simulink model "bounding_spine_Physical"  (R2024a)
settings: Solver=FixedStepDiscrete  StartTime=0.0  StopTime=inf  RelTol=1e-3  EnableMultiTasking=on
InitFcn:
  | run('initBusObjects.m')
  | run('parameters.m')
model workspace (MAT data in the model file):
  omega = 8
  zeta = 0.05
libraries: aru_toolbox x1
settings Model: SimulationMode=external  Creator=Mechatronics  LastModifiedBy=heath
settings SolverCC: ConcurrentTasks=on  AlgebraicLoopSolver=TrustRegion  PositivePriorityOrder=on  InsertRTBMode=Never (minimum delay)
settings DataIOCC: SaveFormat=Array  SaveState=on  SignalLoggingName=logsOut
settings OptimizationCC: BlockReduction=off  BooleanDataType=off  OptimizeBlockIOStorage=off  BufferReuse=off  GlobalBufferReuse=off  ExpressionFolding=off  LocalBlockOutputs=off  InitFltsAndDblsToZero=on  OptimizeDataStoreBuffers=off  BusAssignmentInplaceUpdate=off
settings DebuggingCC: SaveWithParameterizedLinksMsg=none  UnderspecifiedInitializationDetection=Classic  MergeDetectMultiDrivingBlocksExec=none  CheckExecutionContextPreStartOutputMsg=on  SignalResolutionControl=TryResolveAllWithWarning  TasksWithSamePriorityMsg=none  UnconnectedInputMsg=warning  UnconnectedOutputMsg=warning  UnconnectedLineMsg=warning  SFUnexpectedBacktrackingDiag=warning  SFNoUnconditionalDefaultTransitionDiag=warning  SFExecutionAtInitializationDiag=none  ArithmeticOperatorsInVariantConditions=warning
settings HardwareCC: ProdBitPerLong=64  ProdLongLongMode=on  ProdHWDeviceType=Intel->x86-64 (Linux 64)
settings ModelReferenceCC: EnableRefExpFcnMdlSchedulingChecks=on  PropagateSignalLabelsOutOfModel=off
settings SFSimCC: SimUseLocalCustomCode=off  SimTargetLang=C++
settings RTWCC: Description=Speedgoat Real-Time Target Machine  SystemTargetFile=speedgoat.tlc  TemplateMakefile=slrealtime_default_tmf  RTWUseLocalCustomCode=off  Toolchain=Simulink Real-Time Toolchain  BuildConfiguration=Faster Runs  CodeExecutionProfiling=on  TargetLang=C++  GPUComputeCapability=3.5  DLArmComputeVersion=19.05
settings CodeAppCC: StateflowObjectComments=on
settings SimulinkRealTimeTargetCC: InstructionSetFMA=off  LogToMDFFile=off
settings ConfigComp: CovMetricSettings=dw  CovSaveCumulativeToWorkspaceVar=on  CovSaveSingleToWorkspaceVar=on  CovExternalEMLEnable=off  CovSFcnEnable=off

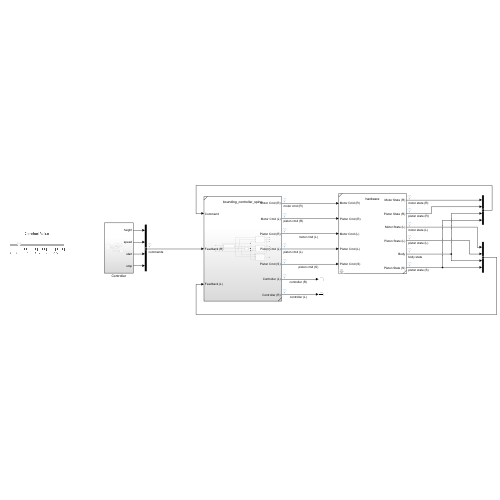
[thumbnail: Simulink's stored preview of the top-level diagram]
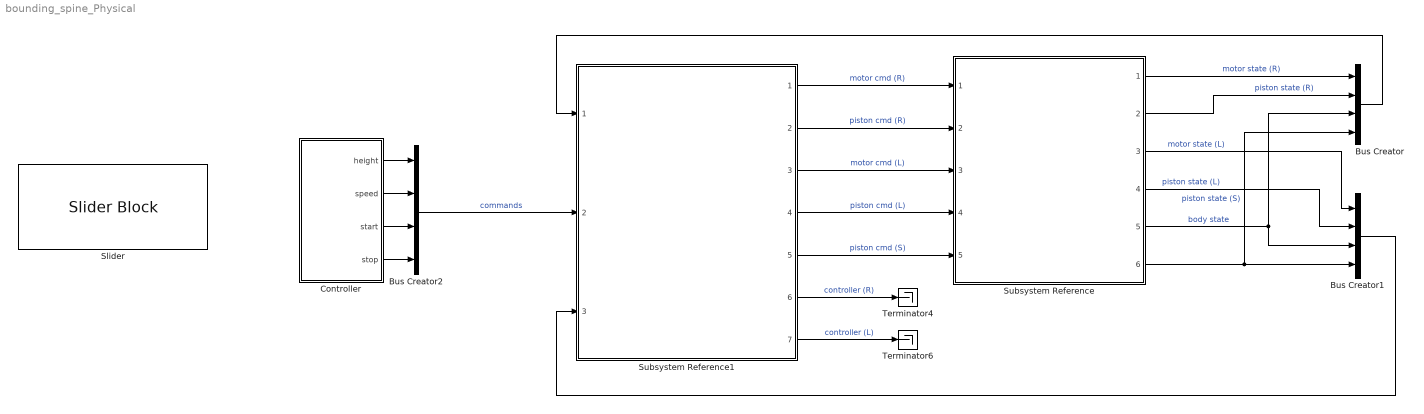
== system bounding_spine_Physical ==
  Bus Creator : BusCreator  Inputs=4  OutDataTypeStr=Bus: State  NonVirtualBus=on
      settings: InheritFromInputs=off
  Bus Creator1 : BusCreator  Inputs=4  OutDataTypeStr=Bus: State  NonVirtualBus=on
      settings: InheritFromInputs=off
  Bus Creator2 : BusCreator  Inputs=4  OutDataTypeStr=Bus: Command  NonVirtualBus=on
      settings: InheritFromInputs=off
  Controller : Subsystem
  Slider : SliderBlock  ScaleMax=3.0
  Subsystem Reference : Subsystem  ReferencedSubsystem=hardware  RollOffset=0
  Subsystem Reference1 : Subsystem  ReferencedSubsystem=bounding_controller_spine
  Terminator4 : Terminator
  Terminator6 : Terminator
  wires:
  Subsystem Reference1/3 -> Subsystem Reference/3  "motor cmd (L)"
  Subsystem Reference/4 -> Bus Creator1/2  "piston state (L)"
  Subsystem Reference/1 -> Bus Creator/1  "motor state (R)"
  Bus Creator1/1 -> Subsystem Reference1/3
  Controller/2(speed) -> Bus Creator2/2
  Subsystem Reference1/7 -> Terminator6/1  "controller (L)"
  Controller/1(height) -> Bus Creator2/1
  Controller/3(start) -> Bus Creator2/3
  Controller/4(stop) -> Bus Creator2/4
  Subsystem Reference1/6 -> Terminator4/1  "controller (R)"
  Bus Creator2/1 -> Subsystem Reference1/2  "commands"
  Bus Creator/1 -> Subsystem Reference1/1
  Subsystem Reference1/4 -> Subsystem Reference/4  "piston cmd (L)"
  Subsystem Reference1/2 -> Subsystem Reference/2  "piston cmd (R)"
  Subsystem Reference1/5 -> Subsystem Reference/5  "piston cmd (S)"
  Subsystem Reference/5 -> Bus Creator1/3, Bus Creator/3  "body state"
  Subsystem Reference/2 -> Bus Creator/2  "piston state (R)"
  Subsystem Reference/3 -> Bus Creator1/1  "motor state (L)"
  Subsystem Reference/6 -> Bus Creator1/4, Bus Creator/4  "piston state (S)"
  Subsystem Reference1/1 -> Subsystem Reference/1  "motor cmd (R)"

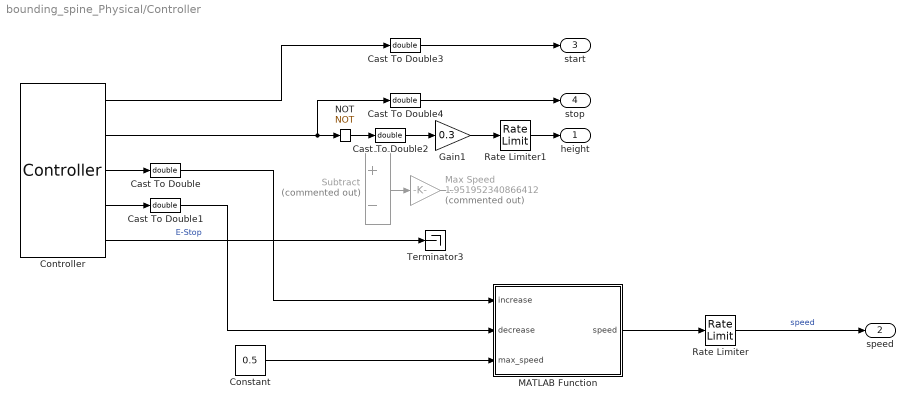
== system bounding_spine_Physical/Controller ==
  Cast To Double{,1..4} (5 alike) : DataTypeConversion  OutDataTypeStr=double  SaturateOnIntegerOverflow=off  RndMeth=Floor
  Constant : Constant  Value=0.5
  Controller : aru_toolbox/Controller
      link override "LVTTL digital input ": parInternalModuleId=1
      settings: SourceProductName=ARU Toolbox
  Gain1 : Gain  Gain=0.3
  MATLAB Function : MATLAB Function  TreatAsAtomicUnit=on
  Max Speed : Gain  Commented=on  Gain=1.951952340866412
  NOT : Logic  Operator=NOT  IconShape=distinctive  AllPortsSameDT=off  OutDataTypeStr=boolean
  Rate Limiter : RateLimiter  RisingSlewLimit=0.15  FallingSlewLimit=-0.15  SampleTimeMode=inherited
  Rate Limiter1 : RateLimiter  RisingSlewLimit=0.05  FallingSlewLimit=-0.05  SampleTimeMode=inherited  InitialCondition=0.26
  Subtract : Sum  Commented=on  Inputs=+-
  Terminator3 : Terminator
  height : Outport
  speed : Outport  Port=2
  start : Outport  Port=3
  stop : Outport  Port=4
  wires:
  Gain1/1 -> Rate Limiter1/1
  Subtract/1 -> Max Speed/1
  Controller/5 -> Terminator3/1  "E-Stop"
  Controller/2 -> Cast To Double4/1, NOT/1
  Controller/3 -> Cast To Double/1
  Max Speed/1 -> ?
  Controller/4 -> Cast To Double1/1
  Cast To Double/1 -> MATLAB Function/1(increase)
  Cast To Double1/1 -> MATLAB Function/2(decrease)
  Controller/1 -> Cast To Double3/1
  Rate Limiter1/1 -> height/1
  Cast To Double3/1 -> start/1
  NOT/1 -> Cast To Double2/1
  Cast To Double2/1 -> Gain1/1
  Cast To Double4/1 -> stop/1
  MATLAB Function/1(speed) -> Rate Limiter/1
  Constant/1 -> MATLAB Function/3(max_speed)
  Rate Limiter/1 -> speed/1  "speed"

== matlab function bounding_spine_Physical/Controller/MATLAB Function ==
  data: increase input; speed output; decrease input; max_speed input
function speed = speed_counter(increase, decrease,max_speed)

persistent count;

if isempty(count)
    count = 0;
end

count = count + increase - decrease;

speed = max(0,min(count,max_speed));
